simulink model "linear_control"  (R2024b)
settings: Solver=ode45  StartTime=0.0  StopTime=100  RelTol=1e-3
values from neighbouring files (symbols this model uses):
  alpha = p(10)    [tumor_growth_controlled.m]    (also in tumor_growth_state_controlled.m)
  b1 = p(3)    [tumor_growth_controlled.m]    (also in tumor_growth_state_controlled.m)
  b2 = p(4)    [tumor_growth_controlled.m]    (also in tumor_growth_state_controlled.m)
  c1 = p(5)    [tumor_growth_controlled.m]    (also in tumor_growth_state_controlled.m)
  c2 = p(6)    [tumor_growth_controlled.m]    (also in tumor_growth_state_controlled.m)
  c3 = p(7)    [tumor_growth_controlled.m]    (also in tumor_growth_state_controlled.m)
  c4 = p(8)    [tumor_growth_controlled.m]    (also in tumor_growth_state_controlled.m)
  d1 = p(12)    [tumor_growth_controlled.m]    (also in tumor_growth_state_controlled.m)
  gamma1 = p(13)    [tumor_growth_controlled.m]    (also in tumor_growth_state_controlled.m)
  gamma2 = p(14)    [tumor_growth_controlled.m]    (also in tumor_growth_state_controlled.m)
  gamma3 = p(15)    [tumor_growth_controlled.m]    (also in tumor_growth_state_controlled.m)
  k = p(16)    [tumor_growth_controlled.m]    (also in tumor_growth_state_controlled.m)
  r1 = p(1)    [tumor_growth_controlled.m]    (also in tumor_growth_state_controlled.m)
  r2 = p(2)    [tumor_growth_controlled.m]    (also in tumor_growth_state_controlled.m)
  rho = p(9)    [tumor_growth_controlled.m]    (also in tumor_growth_state_controlled.m)
  s = p(11)    [tumor_growth_controlled.m]    (also in tumor_growth_state_controlled.m)
undefined symbols (not defined in the file or in its folder): A_int, B_int, C_int, e_init, K_LQ_i, K_LQ_p, x_0, x_eq
settings Model: Creator=fiore  LastModifiedBy=fiore

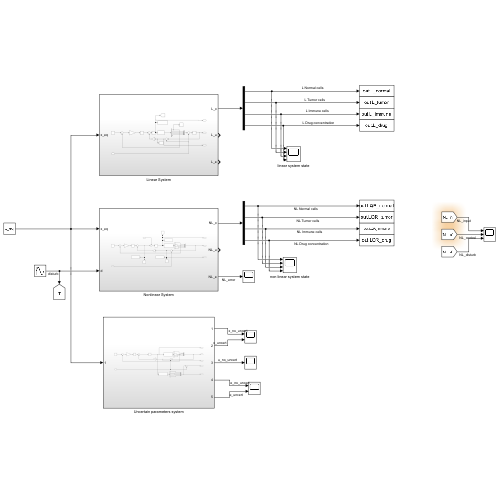
[thumbnail: Simulink's stored preview of the top-level diagram]
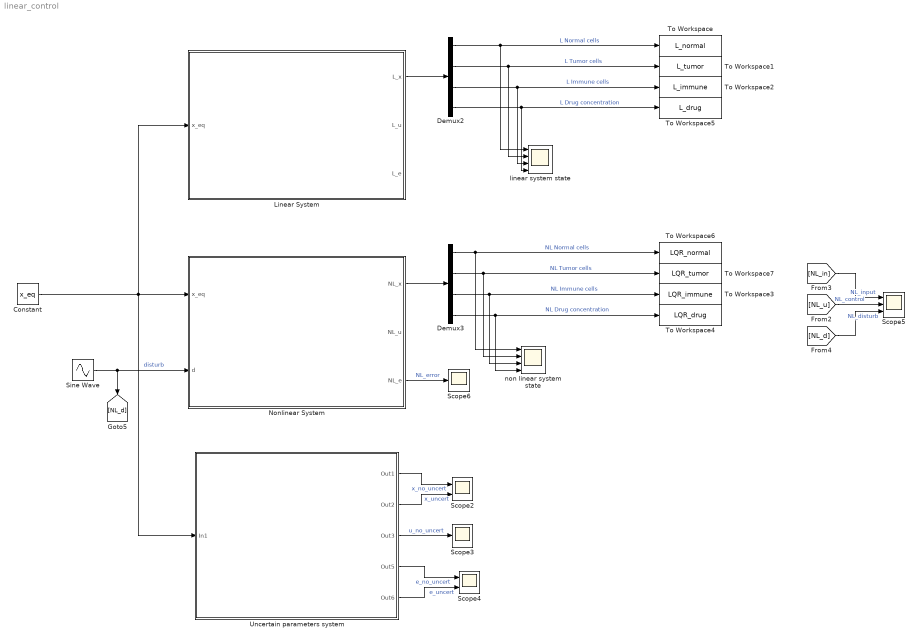
== system linear_control ==
  Constant : Constant  Value=x_eq
  Demux2 : Demux
  Demux3 : Demux
  Linear System : Subsystem
  Nonlinear System : Subsystem
  Scope2 : Scope  NumInputPorts=2
  Scope3 : Scope
  Scope4 : Scope  NumInputPorts=2
  Scope5 : Scope  NumInputPorts=3
  Scope6 : Scope
  Sine Wave : Sin  Amplitude=1.5  Frequency=0.5  SampleTime=0
  To Workspace : ToWorkspace  VariableName=L_normal  SaveFormat=Timeseries  SampleTime=-1
  To Workspace1 : ToWorkspace  VariableName=L_tumor  SaveFormat=Timeseries  SampleTime=-1
  To Workspace2 : ToWorkspace  VariableName=L_immune  SaveFormat=Timeseries  SampleTime=-1
  To Workspace3 : ToWorkspace  VariableName=LQR_immune  SaveFormat=Timeseries  SampleTime=-1
  To Workspace4 : ToWorkspace  VariableName=LQR_drug  SaveFormat=Timeseries  SampleTime=-1
  To Workspace5 : ToWorkspace  VariableName=L_drug  SaveFormat=Timeseries  SampleTime=-1
  To Workspace6 : ToWorkspace  VariableName=LQR_normal  SaveFormat=Timeseries  SampleTime=-1
  To Workspace7 : ToWorkspace  VariableName=LQR_tumor  SaveFormat=Timeseries  SampleTime=-1
  Uncertain parameters system : Subsystem
  linear system state : Scope  NumInputPorts=4
  non linear system state : Scope  NumInputPorts=4
  wires:
  Demux2/1 -> To Workspace/1, linear system state/1  "L Normal cells"
  Demux2/2 -> To Workspace1/1, linear system state/2  "L Tumor cells"
  Demux2/3 -> To Workspace2/1, linear system state/3  "L Immune cells"
  Demux2/4 -> To Workspace5/1, linear system state/4  "L Drug concentration"
  Demux3/4 -> To Workspace4/1, non linear system state/4  "NL Drug concentration"
  Demux3/1 -> To Workspace6/1, non linear system state/1  "NL Normal cells"
  Demux3/2 -> To Workspace7/1, non linear system state/2  "NL Tumor cells"
  Demux3/3 -> To Workspace3/1, non linear system state/3  "NL Immune cells"
  [NL_in] -> Scope5/1  "NL_input"
  [NL_u] -> Scope5/2  "NL_control"
  [NL_d] -> Scope5/3  "NL_disturb"
  Uncertain parameters system/1(Out1) -> Scope2/1  "x_no_uncert"
  Uncertain parameters system/2(Out2) -> Scope2/2  "x_uncert"
  Uncertain parameters system/3(Out3) -> Scope3/1  "u_no_uncert"
  Uncertain parameters system/4(Out5) -> Scope4/1  "e_no_uncert"
  Uncertain parameters system/5(Out6) -> Scope4/2  "e_uncert"
  Linear System/1(L_x) -> Demux2/1
  Nonlinear System/1(NL_x) -> Demux3/1
  Constant/1 -> Uncertain parameters system/1(In1), Linear System/1(x_eq), Nonlinear System/1(x_eq)
  Nonlinear System/3(NL_e) -> Scope6/1  "NL_error"
  Sine Wave/1 -> Nonlinear System/2(d), [NL_d]  "disturb"

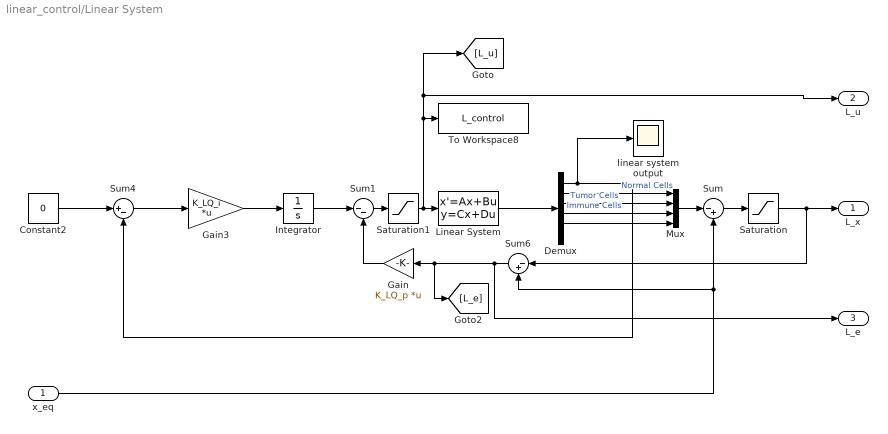
== system linear_control/Linear System ==
  x_eq : Inport
  Constant2 : Constant  Value=0
  Demux : Demux  Outputs=6
  Gain : Gain  Gain=K_LQ_p  Multiplication=Matrix(K*u)
  Gain3 : Gain  Gain=K_LQ_i  Multiplication=Matrix(K*u)
  Integrator : Integrator
  Linear System : StateSpace  A=A_int  B=B_int  C=[C_int;eye(5)]  D=[0,0,0,0,0,0]'  InitialCondition=e_init
  Mux : Mux
  Saturation : Saturate  UpperLimit=100  LowerLimit=0
  Saturation1 : Saturate  UpperLimit=0  LowerLimit=-100
  Sum : Sum  Inputs=|-+
  Sum1 : Sum  Inputs=|--
  Sum4 : Sum  Inputs=|+-
  Sum6 : Sum  Inputs=|-+
  To Workspace8 : ToWorkspace  VariableName=L_control  SaveFormat=Timeseries  SampleTime=-1
  linear system output : Scope
  L_x : Outport
  L_u : Outport  Port=2
  L_e : Outport  Port=3
  wires:
  Constant2/1 -> Sum4/1
  Sum1/1 -> Saturation1/1
  Sum6/1 -> [L_e], Gain/1, L_e/1
  Linear System/1 -> Demux/1
  Sum4/1 -> Gain3/1
  Demux/4 -> Mux/3  "Immune Cells"
  Saturation/1 -> L_x/1, Sum6/1
  Integrator/1 -> Sum1/1
  x_eq/1 -> Sum/2, Sum6/2
  Mux/1 -> Sum/1
  Demux/1 -> linear system output/1, Sum4/2
  Demux/2 -> Mux/1  "Normal Cells"
  Demux/3 -> Mux/2  "Tumor Cells"
  Demux/5 -> Mux/4
  Gain/1 -> Sum1/2
  Gain3/1 -> Integrator/1
  Sum/1 -> Saturation/1
  Saturation1/1 -> L_u/1, [L_u], To Workspace8/1, Linear System/1

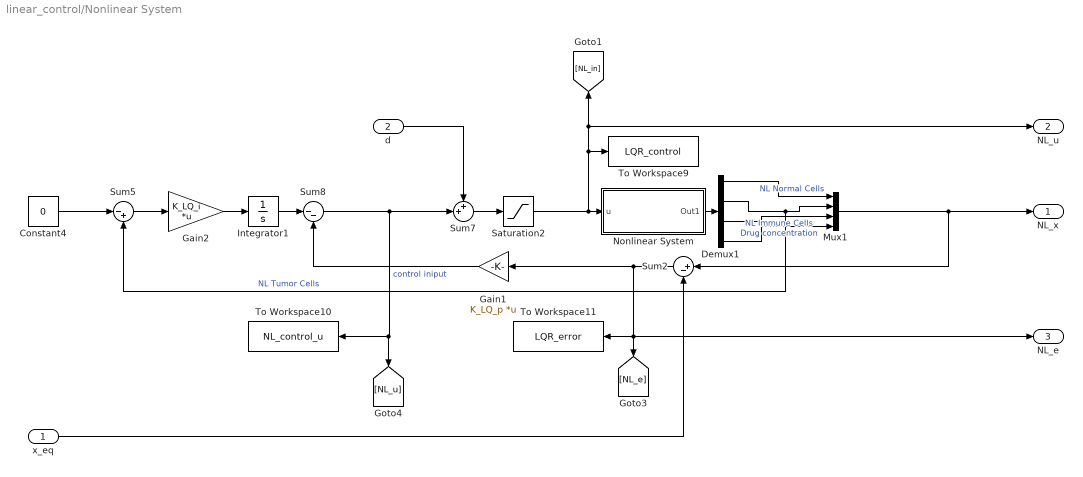
== system linear_control/Nonlinear System ==
  x_eq : Inport
  d : Inport  Port=2
  Constant4 : Constant  Value=0
  Demux1 : Demux
  Gain1 : Gain  Gain=K_LQ_p  Multiplication=Matrix(K*u)
  Gain2 : Gain  Gain=K_LQ_i  Multiplication=Matrix(K*u)
  Integrator1 : Integrator
  Mux1 : Mux
  Nonlinear System : Subsystem
  Saturation2 : Saturate  UpperLimit=inf  LowerLimit=0  ZeroCross=off
  Sum2 : Sum  Inputs=|+-
  Sum5 : Sum  Inputs=|-+
  Sum7 : Sum  Inputs=++|
  Sum8 : Sum  Inputs=|--
  To Workspace10 : ToWorkspace  VariableName=NL_control_u  SaveFormat=Timeseries  SampleTime=-1
  To Workspace11 : ToWorkspace  VariableName=LQR_error  SaveFormat=Timeseries  SampleTime=-1
  To Workspace9 : ToWorkspace  VariableName=LQR_control  SaveFormat=Timeseries  SampleTime=-1
  NL_x : Outport
  NL_u : Outport  Port=2
  NL_e : Outport  Port=3
  wires:
  Saturation2/1 -> [NL_in], NL_u/1, To Workspace9/1, Nonlinear System/1(u)
  Sum2/1 -> NL_e/1, [NL_e], To Workspace11/1, Gain1/1
  Gain2/1 -> Integrator1/1
  Sum7/1 -> Saturation2/1
  Demux1/2 -> Mux1/2, Sum5/2  "NL Tumor Cells"
  Mux1/1 -> NL_x/1, Sum2/1
  Sum8/1 -> Sum7/2, [NL_u], To Workspace10/1  "control iniput"
  Integrator1/1 -> Sum8/1
  x_eq/1 -> Sum2/2
  Sum5/1 -> Gain2/1
  Constant4/1 -> Sum5/1
  Demux1/1 -> Mux1/1  "NL Normal Cells"
  Gain1/1 -> Sum8/2
  Demux1/3 -> Mux1/3  "NL Immune Cells"
  Nonlinear System/1(Out1) -> Demux1/1
  Demux1/4 -> Mux1/4  "Drug concentration"
  d/1 -> Sum7/1

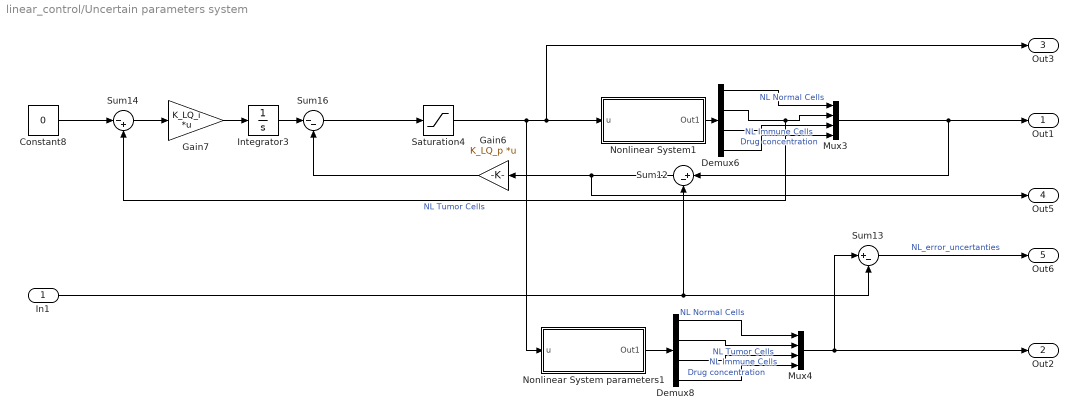
== system linear_control/Uncertain parameters system ==
  In1 : Inport
  Constant8 : Constant  Value=0
  Demux6 : Demux
  Demux8 : Demux
  Gain6 : Gain  Gain=K_LQ_p  Multiplication=Matrix(K*u)
  Gain7 : Gain  Gain=K_LQ_i  Multiplication=Matrix(K*u)
  Integrator3 : Integrator
  Mux3 : Mux
  Mux4 : Mux
  Nonlinear System parameters1 : Subsystem
  Nonlinear System1 : Subsystem
  Saturation4 : Saturate  UpperLimit=inf  LowerLimit=0
  Sum12 : Sum  Inputs=|+-
  Sum13 : Sum  Inputs=|+-
  Sum14 : Sum  Inputs=|-+
  Sum16 : Sum  Inputs=|--
  Out1 : Outport
  Out2 : Outport  Port=2
  Out3 : Outport  Port=3
  Out5 : Outport  Port=4
  Out6 : Outport  Port=5
  wires:
  Demux8/4 -> Mux4/4  "Drug concentration"
  Sum16/1 -> Saturation4/1
  Demux8/2 -> Mux4/2  "NL Tumor Cells"
  Demux6/2 -> Mux3/2, Sum14/2  "NL Tumor Cells"
  Demux6/1 -> Mux3/1  "NL Normal Cells"
  Demux6/4 -> Mux3/4  "Drug concentration"
  Integrator3/1 -> Sum16/1
  Sum14/1 -> Gain7/1
  Nonlinear System1/1(Out1) -> Demux6/1
  Sum13/1 -> Out6/1  "NL_error_uncertanties"
  Sum12/1 -> Out5/1, Gain6/1
  Gain6/1 -> Sum16/2
  Gain7/1 -> Integrator3/1
  Demux6/3 -> Mux3/3  "NL Immune Cells"
  Mux4/1 -> Out2/1, Sum13/1
  Constant8/1 -> Sum14/1
  In1/1 -> Sum13/2, Sum12/2
  Saturation4/1 -> Out3/1, Nonlinear System1/1(u), Nonlinear System parameters1/1(u)
  Mux3/1 -> Sum12/1, Out1/1
  Demux8/1 -> Mux4/1  "NL Normal Cells"
  Demux8/3 -> Mux4/3  "NL Immune Cells"
  Nonlinear System parameters1/1(Out1) -> Demux8/1

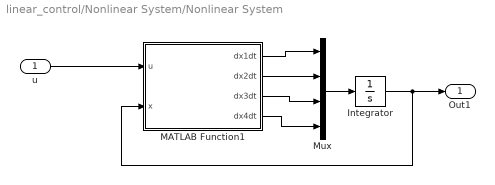
== system linear_control/Nonlinear System/Nonlinear System ==
  u : Inport
  Integrator : Integrator  InitialCondition=x_0  LimitOutput=on  UpperSaturationLimit=+inf  LowerSaturationLimit=0
  MATLAB Function1 : MATLAB Function  TreatAsAtomicUnit=on
  Mux : Mux
  Out1 : Outport
  wires:
  MATLAB Function1/2(dx2dt) -> Mux/2
  MATLAB Function1/1(dx1dt) -> Mux/1
  MATLAB Function1/3(dx3dt) -> Mux/3
  Mux/1 -> Integrator/1
  Integrator/1 -> Out1/1, MATLAB Function1/2(x)
  u/1 -> MATLAB Function1/1(u)
  MATLAB Function1/4(dx4dt) -> Mux/4

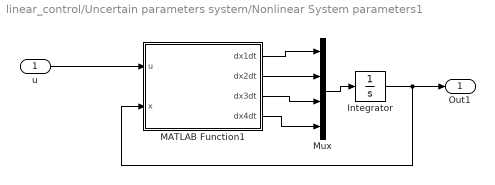
== system linear_control/Uncertain parameters system/Nonlinear System parameters1 ==
  u : Inport
  Integrator : Integrator  InitialCondition=x_0  LimitOutput=on  UpperSaturationLimit=+inf  LowerSaturationLimit=0
  MATLAB Function1 : MATLAB Function  TreatAsAtomicUnit=on
  Mux : Mux
  Out1 : Outport
  wires:
  MATLAB Function1/2(dx2dt) -> Mux/2
  MATLAB Function1/1(dx1dt) -> Mux/1
  MATLAB Function1/3(dx3dt) -> Mux/3
  Mux/1 -> Integrator/1
  Integrator/1 -> MATLAB Function1/2(x), Out1/1
  u/1 -> MATLAB Function1/1(u)
  MATLAB Function1/4(dx4dt) -> Mux/4

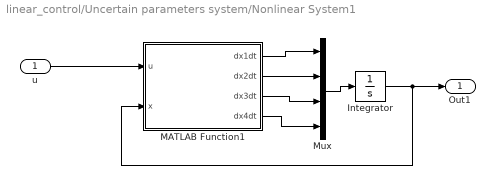
== system linear_control/Uncertain parameters system/Nonlinear System1 ==
  u : Inport
  Integrator : Integrator  InitialCondition=x_0  LimitOutput=on  UpperSaturationLimit=+inf  LowerSaturationLimit=0
  MATLAB Function1 : MATLAB Function  TreatAsAtomicUnit=on
  Mux : Mux
  Out1 : Outport
  wires:
  MATLAB Function1/2(dx2dt) -> Mux/2
  MATLAB Function1/1(dx1dt) -> Mux/1
  MATLAB Function1/3(dx3dt) -> Mux/3
  Mux/1 -> Integrator/1
  Integrator/1 -> MATLAB Function1/2(x), Out1/1
  u/1 -> MATLAB Function1/1(u)
  MATLAB Function1/4(dx4dt) -> Mux/4

== matlab function linear_control/Nonlinear System/Nonlinear System/MATLAB Function1 ==
  data: u input; dx1dt output; x input; dx2dt output; r1 parameter; r2 parameter; b1 parameter; b2 parameter; c1 parameter; c3 parameter; c2 parameter; c4 parameter; rho parameter; alpha parameter; s parameter; d1 parameter; dx3dt output; gamma1 parameter; gamma2 parameter; gamma3 parameter; dx4dt output; k parameter
function [dx1dt,dx2dt,dx3dt, dx4dt] = tumor_growth(u,x,r1, r2, b1, b2, c1, c3, c2, c4, rho, alpha, s, d1, gamma1, gamma2, gamma3, k)

    x1 = x(1);       % (normal cells)
    x2 = x(2);       % (tumor cells)
    x3 = x(3);       % (immune cells)
    x4 = x(4);       % (drug concentration)
    
    dx1dt = r2 * x1 * (1 - b2 * x1) - c4 * x2 * x1 - gamma1 * x4;
    dx2dt = r1 * x2 * (1 - b1 * x2) - c2 * x3 * x2 - c3 * x2 * x1 - gamma2 * x4;
    dx3dt = s + (rho * x3 * x2) / (alpha + x2) - c1 * x3 * x2 - d1 * x3 - gamma3 * x4;   
    dx4dt = u - k*x4;
end

== matlab function linear_control/Uncertain parameters system/Nonlinear System parameters1/MATLAB Function1 ==
  data: u input; dx1dt output; x input; dx2dt output; r1 parameter; r2 parameter; b1 parameter; b2 parameter; c1 parameter; c3 parameter; c2 parameter; c4 parameter; rho parameter; alpha parameter; s parameter; d1 parameter; dx3dt output; gamma1 parameter; gamma2 parameter; gamma3 parameter; dx4dt output; k parameter
function [dx1dt,dx2dt,dx3dt, dx4dt] = tumor_growth(u,x,r1, r2, b1, b2, c1, c3, c2, c4, rho, alpha, s, d1, gamma1, gamma2, gamma3, k)

    c1_real = c1*(1-0.5);
    c4_real = c4*(1-0.5);

    x1 = x(1);       % (normal cells)
    x2 = x(2);       % (tumor cells)
    x3 = x(3);       % (immune cells)
    x4 = x(4);       % (drug concentration)
    
    dx1dt = r2 * x1 * (1 - b2 * x1) - c4_real * x2 * x1 - gamma1 * x4;
    dx2dt = r1 * x2 * (1 - b1 * x2) - c2 * x3 * x2 - c3 * x2 * x1 - gamma2 * x4;
    dx3dt = s + (rho * x3 * x2) / (alpha + x2) - c1_real * x3 * x2 - d1 * x3 - gamma3 * x4;   
    dx4dt = u - k*x4;
end

== matlab function linear_control/Uncertain parameters system/Nonlinear System1/MATLAB Function1 ==
  data: u input; dx1dt output; x input; dx2dt output; r1 parameter; r2 parameter; b1 parameter; b2 parameter; c1 parameter; c3 parameter; c2 parameter; c4 parameter; rho parameter; alpha parameter; s parameter; d1 parameter; dx3dt output; gamma1 parameter; gamma2 parameter; gamma3 parameter; dx4dt output; k parameter
function [dx1dt,dx2dt,dx3dt, dx4dt] = tumor_growth(u,x,r1, r2, b1, b2, c1, c3, c2, c4, rho, alpha, s, d1, gamma1, gamma2, gamma3, k)

    x1 = x(1);       % (normal cells)
    x2 = x(2);       % (tumor cells)
    x3 = x(3);       % (immune cells)
    x4 = x(4);       % (drug concentration)
    
    dx1dt = r2 * x1 * (1 - b2 * x1) - c4 * x2 * x1 - gamma1 * x4;
    dx2dt = r1 * x2 * (1 - b1 * x2) - c2 * x3 * x2 - c3 * x2 * x1 - gamma2 * x4;
    dx3dt = s + (rho * x3 * x2) / (alpha + x2) - c1 * x3 * x2 - d1 * x3 - gamma3 * x4;   
    dx4dt = u - k*x4;
end
